simulink model "simulation"  (R2020a)
settings: Solver=ode23t  StartTime=0.0  StopTime=50  MaxStep=0.5  MinStep=1e-10  RelTol=1  EnableMultiTasking=on
libraries: simulink x1, powerlib x1
settings Model: Creator=Green  LastModifiedBy=Catherine Cai
settings SolverCC: MaxConsecutiveMinStep=5
settings DataIOCC: LimitDataPoints=on  SaveFormat=Array  SignalLoggingSaveFormat=ModelDataLogs  ReturnWorkspaceOutputs=off
settings OptimizationCC: ExpressionDepthLimit=2147483647  LifeSpan=inf
settings DebuggingCC: UnderspecifiedInitializationDetection=Classic  MergeDetectMultiDrivingBlocksExec=none  FcnCallInpInsideContextMsg=warning  StateNameClashWarn=warning  SFUnexpectedBacktrackingDiag=warning  SFNoUnconditionalDefaultTransitionDiag=warning  SFExecutionAtInitializationDiag=none  ArithmeticOperatorsInVariantConditions=warning
settings HardwareCC: ProdBitPerPointer=32  ProdBitPerSizeT=32  ProdBitPerPtrDiffT=32  ProdLargestAtomicFloat=None  ProdIntDivRoundTo=Undefined  ProdEndianess=Unspecified  ProdWordSize=32  ProdHWDeviceType=32-bit Generic
settings ModelReferenceCC: PropagateSignalLabelsOutOfModel=off
settings SFSimCC: SimUseLocalCustomCode=off  CustomCodeUndefinedFunction=UseInterfaceOnly
settings RTWCC: RTWUseLocalCustomCode=off
settings CodeAppCC: StateflowObjectComments=on
settings GRTTargetCC: TargetLangStandard=C89/C90 (ANSI)  CombineOutputUpdateFcns=off  GRTInterface=on
settings ConfigComp: CovMetricSettings=dw  CovSaveCumulativeToWorkspaceVar=on  CovSaveSingleToWorkspaceVar=on  CovExternalEMLEnable=off
settings SimscapeCC: SimscapeNormalizeSystem=off

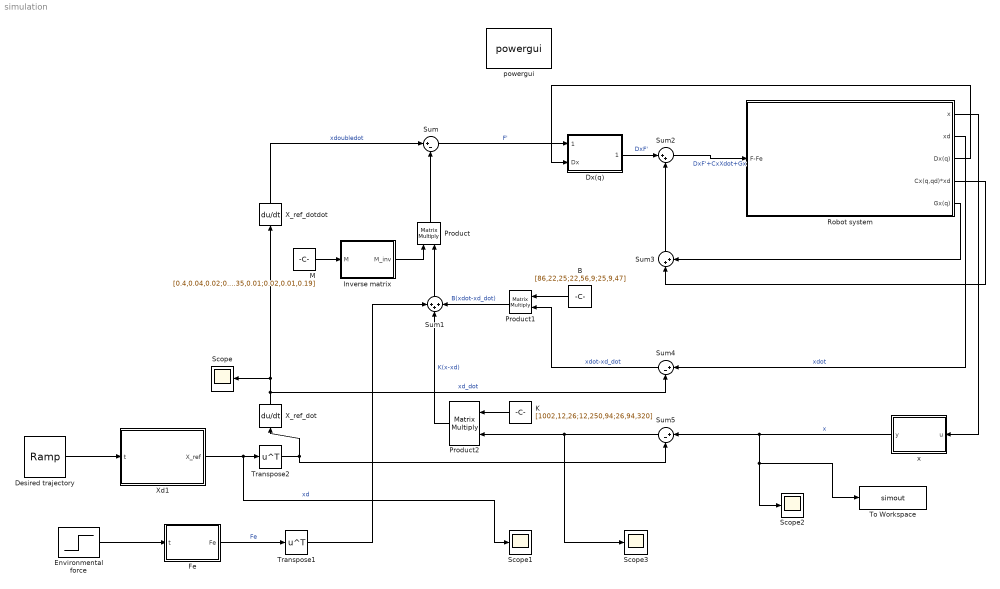
== system simulation ==
  B : Constant  Value=[86,22,25;22,56,9;25,9,47]  VectorParams1D=off
  Desired trajectory : simulink/Sources/Ramp  slope=0.1  start=0  InitialOutput=0
  Dx(q) : MATLAB Function  TreatAsAtomicUnit=on
  Environmental force : Step  SampleTime=0
  Fe : MATLAB Function  TreatAsAtomicUnit=on
  Inverse matrix : MATLAB Function  TreatAsAtomicUnit=on
  K : Constant  Value=[1002,12,26;12,250,94;26,94,320]  VectorParams1D=off
  M : Constant  Value=[0.4,0.04,0.02;0.03,0.035,0.01;0.02,0.01,0.19]  VectorParams1D=off
  Product : Product  Multiplication=Matrix(*)
  Product1 : Product  Multiplication=Matrix(*)
  Product2 : Product  Multiplication=Matrix(*)
  Robot system : Subsystem
  Scope{,1..3} (4 alike) : Scope
  Sum : Sum  Inputs=|+-
  Sum1 : Sum  Inputs=+++
  Sum2 : Sum  Inputs=|++
  Sum3 : Sum  Inputs=|++
  Sum4 : Sum  Inputs=|+-
  Sum5 : Sum  Inputs=|+-
  To Workspace : ToWorkspace  VariableName=simout  SaveFormat=Timeseries  SampleTime=-1
  Transpose1 : Math  Operator=transpose  SaturateOnIntegerOverflow=on
  Transpose2 : Math  Operator=transpose  SaturateOnIntegerOverflow=on
  X_ref_dot : Derivative
  X_ref_dotdot : Derivative
  Xd1 : MATLAB Function  TreatAsAtomicUnit=on
  powergui : powerlib/powergui  Priority=1  SimulationMode=Discrete  SampleTime=50e-8  frequency=60  Iterations=50  frequencyindice=60  Pbase=100e6  ErrMax=1e-4  UnitsV=kV  UnitsW=MW  buscounter=0  FunctionMessages=off  echomessages=off  EnableUseOfTLC=off  CurrentSourceSwitches=off  DisableSnubberDevices=off  DisableRonSwitches=off  DisableVfSwitches=off  DisplayEquations=off  AutomaticDiscreteSolvers=off  SolverType=Tustin/Backward Euler (TBE)  Interpol=off  ExternalGateDelay=off  methode=off  Ts=100  x0status=blocks  SPID=off  SwTol=0  HookPort=off  NonlinearTolerance=1e-4  nMaxIteration=100  ContinueOnMaxIteration=off  RestoreLinks=warning  ResistiveCurrentMeasurement=off  Frange=[0:2:500]  Ylog=off  Xlog=on  ShowGrid=off  save=off  variable=ZData  structure=0  ZoomFFT=off  StartTime=0.0  cycles=1  DisplayStyle=1  fundamental=60  FreqAxis=off  MaxFrequency=1000  frequencyindicesteady=1  RmsSteady=1  display=off
  x : MATLAB Function  TreatAsAtomicUnit=on
  wires:
  Product/1 -> Sum/2
  Sum1/1 -> Product/2
  X_ref_dot/1 -> X_ref_dotdot/1, Scope/1, Sum4/2  "xd_dot"
  X_ref_dotdot/1 -> Sum/1  "xdoubledot"
  Sum/1 -> Dx(q)/1(F_prime)  "F'"
  Dx(q)/1(Dx_Fprime) -> Sum2/1  "DxF'"
  Sum2/1 -> Robot system/1(F-Fe)  "DxF'+CxXdot+Gx"
  Sum3/1 -> Sum2/2
  Robot system/2(xd) -> Sum4/1  "xdot"
  Sum4/1 -> Product1/2  "xdot-xd_dot"
  x/1(y) -> To Workspace/1, Scope2/1, Sum5/1  "x"
  Sum5/1 -> Scope3/1, Product2/2
  Inverse matrix/1(M_inv) -> Product/1
  B/1 -> Product1/1
  Product1/1 -> Sum1/3  "B(xdot-xd_dot)"
  K/1 -> Product2/1
  Product2/1 -> Sum1/2  "K(x-xd)"
  Environmental force/1 -> Fe/1(t)
  Transpose1/1 -> Sum1/1
  Fe/1(Fe) -> Transpose1/1  "Fe"
  Xd1/1(X_ref) -> Scope1/1, Transpose2/1  "xd"
  Transpose2/1 -> X_ref_dot/1, Sum5/2
  Robot system/5(Gx(q)) -> Sum3/2
  Robot system/4(Cx(q,qd)*xd) -> Sum3/1
  Robot system/3(Dx(q)) -> Dx(q)/2(Dx)
  Robot system/1(x) -> x/1(u)
  M/1 -> Inverse matrix/1(M)
  Desired trajectory/1 -> Xd1/1(t)

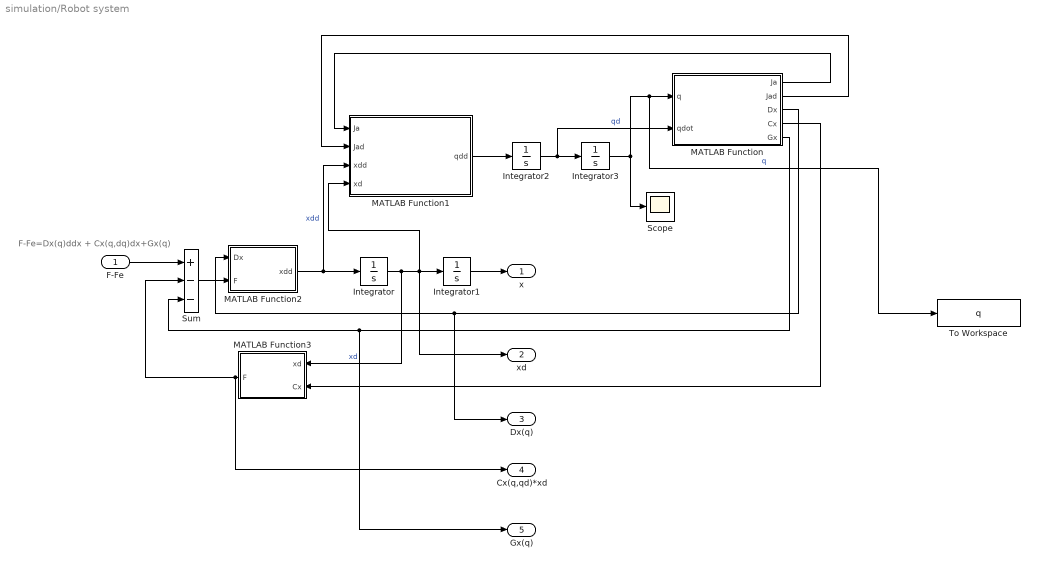
== system simulation/Robot system ==
  note: F-Fe=Dx(q)ddx + Cx(q,dq)dx+Gx(q)
  F-Fe : Inport
  Integrator : Integrator  InitialCondition=[0 0 0]'
  Integrator1 : Integrator  InitialCondition=[0 0 0]'
  Integrator2 : Integrator  InitialCondition=[0 0 0]'
  Integrator3 : Integrator  InitialCondition=[0.1 0.1 0.1]'
  MATLAB Function : MATLAB Function  TreatAsAtomicUnit=on
  MATLAB Function1 : MATLAB Function  TreatAsAtomicUnit=on
  MATLAB Function2 : MATLAB Function  TreatAsAtomicUnit=on
  MATLAB Function3 : MATLAB Function  TreatAsAtomicUnit=on
  Scope : Scope
  Sum : Sum  Inputs=+--
  To Workspace : ToWorkspace  VariableName=q  SaveFormat=Timeseries  SampleTime=-1
  x : Outport
  xd : Outport  Port=2
  Dx(q) : Outport  Port=3
  Cx(q,qd)*xd : Outport  Port=4
  Gx(q) : Outport  Port=5
  wires:
  Sum/1 -> MATLAB Function2/2(F)
  Integrator3/1 -> To Workspace/1, MATLAB Function/1(q), Scope/1  "q"
  MATLAB Function/3(Dx) -> Dx(q)/1, MATLAB Function2/1(Dx)
  MATLAB Function2/1(xdd) -> MATLAB Function1/3(xdd), Integrator/1  "xdd"
  MATLAB Function1/1(qdd) -> Integrator2/1
  MATLAB Function/5(Gx) -> Gx(q)/1, Sum/3
  Integrator1/1 -> x/1
  Integrator/1 -> MATLAB Function3/1(xd), xd/1, MATLAB Function1/4(xd), Integrator1/1  "xd"
  Integrator2/1 -> MATLAB Function/2(qdot), Integrator3/1  "qd"
  MATLAB Function/1(Ja) -> MATLAB Function1/1(Ja)
  MATLAB Function/2(Jad) -> MATLAB Function1/2(Jad)
  MATLAB Function/4(Cx) -> MATLAB Function3/2(Cx)
  MATLAB Function3/1(F) -> Cx(q,qd)*xd/1, Sum/2
  F-Fe/1 -> Sum/1

== matlab function simulation/Robot system/MATLAB Function ==
  data: Ja output; Jad output; q input; Dx output; Cx output; Gx output; qdot input
function [Ja,Jad,Dx,Cx,Gx] = jacobian_cal(q, qdot)
    q1 = q(1);
    q2 = q(2);
    q3 = q(3);
    qd1 = qdot(1);
    qd2 = qdot(2);
    qd3 = qdot(3);

    % Parameters
    m1 = 3.92; %kg
    m2 = 2.16;
    m3 = 1;

    % link length

    l1 = 0.4; % meter
    l2 = 0.3;
    l3 = 0.2;
    
    g = 9.8;
    
    % inertia tensor
    Ic1xx = 0.0587; % kg*meter^2
    Ic1yy = 0.0128;
    Ic1zz = 0.0587;

    Ic2xx = 0.0052;
    Ic2yy = 0.0188;
    Ic2zz = 0.0188;

    Ic3xx = 0.0016;
    Ic3yy = 0.0042;
    Ic3zz = 0.0042;


    % Dq
    q23 = q2+q3;
    d11 = Ic1yy + m2*l2^2*cos(q2)^2/4 + Ic2xx*sin(q2)^2 + ...
          Ic2yy*cos(q2)^2 + m3*l2^2*cos(q2)^2 + m3*l3^2*cos(q23)^2/4 + ...
          m3*l2*l3*cos(q2)*cos(q23)+ Ic3xx*sin(q23)^2 + Ic3yy*cos(q23)^2;

    d22 = m2*l2^2/4 + Ic2zz + m3*l2^2 +...
          m3*l3^2/4 + m3*l2*l3*cos(q3) + Ic3zz;
    d23 = m3*l3^2/4 + m3*l2*l3*cos(q3)/2 + Ic3zz;
    d33 = m3*l3^2/4 + Ic3zz;
    Dq  = [d11,   0,   0;
           0,   d22, d23;
           0,   d23, d33];

    % Cq
    h1 = sin(q2+q2)*(-m2*l2^2/4 + Ic2xx -Ic2yy - m3*l2^2) + ...
         sin(q2*2+q3*2)*(-m3*l3^2/4 + Ic3xx - Ic3yy) - sin(q2+q2+q3)*m3*l2*l3;
    h2 = sin(q2*2+q3*2)*(-m3*l3^2/4 + Ic3xx - Ic3yy) - cos(q2)*sin(q23)*m3*l2*l3;
    h3 = -sin(q3)*m3*l2*l3;
    Cq = 0.5*[h1*qd2 + h2*qd3,  h1*qd1, h2*qd1;
                     - h1*qd1,  h3*qd3, h3*qd2 + h3*qd3;
                     - h2*qd1, -h3*qd2, 0];
    % Gq
    Gq = [ 0;
          -m2*g*l2*cos(q2)/2 - m3*g*l2*cos(q2) - m3*g*l3*cos(q23)/2;
          -m3*g*l3*cos(q23)/2];

    % Analytical Jacobian
    j11 = -l2*sin(q1)*cos(q2)-l3*sin(q1)*cos(q23);
    j12 = -l2*cos(q1)*sin(q2)-l3*cos(q1)*sin(q23);
    j13 = -l3*cos(q1)*sin(q23);
    j21 = l2*cos(q1)*cos(q2)+l3*cos(q1)*cos(q23);
    j22 = -l2*sin(q1)*sin(q2)-l3*sin(q1)*cos(q23);
    j23 = -l3*sin(q1)*sin(q23);
    j31 = 0;
    j32 = -l2*cos(q2)-l3*cos(q23);
    j33 = -3*cos(q23);
    Ja = [j11, j12, j13;
          j21, j22, j23;
          j31, j32, j33];

    % Analytical jacobian dot
    jd11 = -l2*cos(q1)*cos(q2)*qd1   + l2*sin(q1)*sin(q2)*qd2 ...
           - l3*cos(q1)*cos(q23)*qd1 + l3*sin(q1)*sin(q23)*(qd2+qd3);
    jd12 = l2*sin(q1)*sin(q2)*qd1    - l2*cos(q1)*cos(q2)*qd2...
           + l3*sin(q1)*sin(q23)*qd1 - l3*cos(q1)*cos(q23)*(qd2+qd3);
    jd13 = l3*sin(q1)*sin(q23)*qd1   - l3*cos(q1)*cos(q23)*(qd2+qd3);
    jd21 = - l2*sin(q1)*cos(q2)*qd1  - l2*cos(q1)*sin(q2)*qd2...
           - l3*sin(q1)*cos(q23)*qd1 - l3*cos(q1)*sin(q23)*(qd2+qd3);
    jd22 = -l2*cos(q1)*sin(q2)*qd1   - l2*sin(q1)*cos(q2)*qd2...
           - l3*cos(q1)*sin(q23)*qd1 - l3*sin(q1)*cos(q23)*(qd2+qd3);
    jd23 = -l3*cos(q1)*sin(q23)*qd1  - l3*sin(q1)*cos(q23)*(qd2+qd3);
    jd31 = 0;
    jd32 = l2*sin(q2)*qd2 + l3*sin(q23)*(qd2+qd3);
    jd33 = l3*sin(q23)*(qd2+qd3);
    Jad  = [ jd11, jd12, jd13;
             jd21, jd22, jd23;
             jd31, jd32, jd33];
    % inverse transpose     
    Jait = inv(Ja)';
    Dx = Jait*Dq/Ja;
    Cx = Jait*(Cq - Dq/Ja*Jad)/Ja;
    Gx = Jait*Gq;

== matlab function simulation/Dx(q) ==
  data: F_prime input; Dx_Fprime output; Dx input
function Dx_Fprime = fcn(F_prime, Dx)

Dx_Fprime = Dx*F_prime;

== matlab function simulation/Robot system/MATLAB Function1 ==
  data: Ja input; Jad input; xdd input; qdd output; xd input
function qdd = qdoubledot(Ja,Jad,xdd,xd)
qdd = inv(Ja)*xdd - inv(Ja)*Jad*inv(Ja)*xd;

== matlab function simulation/Robot system/MATLAB Function2 ==
  data: Dx input; xdd output; F input
function xdd = fcn(Dx,F)
xdd = inv(Dx)*F;

== matlab function simulation/Robot system/MATLAB Function3 ==
  data: xd input; F output; Cx input
function F = fcn(xd,Cx)

F=Cx*xd;

== matlab function simulation/Xd1 ==
  data: t input; X_ref output
function X_ref  = fcn(t)

x_ref = 0.1 + 0.05 * t;% + 0.1*sin(7*t);
y_ref = 0.3 - 0.05*t;
z_ref = 0.5 + 0.05*t;

X_ref = [x_ref,y_ref,z_ref];

== matlab function simulation/x ==
  data: u input; y output
function y = fcn(u)

y = u;

== matlab function simulation/Fe ==
  data: t input; Fe output
function Fe = fcn(t)

Fe_x = 0.1 + 0.05*t;
Fe_y = 0.3 - 0.05*t;
Fe_z = 0.5 + 0.05*t;

Fe = [Fe_x, Fe_y, Fe_z];

== matlab function simulation/Inverse matrix ==
  data: M input; M_inv output
function M_inv = fcn(M)

M_inv = inv(M);
